simulink model "Toy_example"  (R2024b)
settings: Solver=VariableStepAuto  StartTime=0.0  StopTime=10.0  RelTol=1e-3
settings Model: Creator=Stefania  LastModifiedBy=Stefania

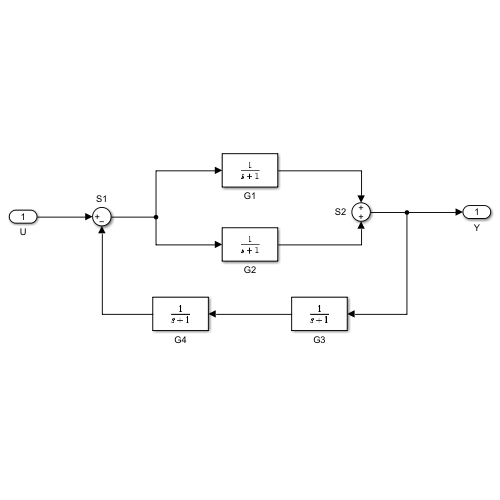
[thumbnail: Simulink's stored preview of the top-level diagram]
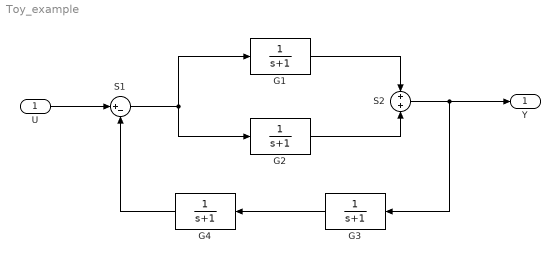
== system Toy_example ==
  U : Inport
  G{1..4} (4 alike) : TransferFcn  Denominator=[1 1]
  S1 : Sum  Inputs=|+-
  S2 : Sum
  Y : Outport
  wires:
  S2/1 -> Y/1, G3/1
  G1/1 -> S2/1
  G2/1 -> S2/2
  S1/1 -> G2/1, G1/1
  G3/1 -> G4/1
  G4/1 -> S1/2
  U/1 -> S1/1
